simulink model "Aenea_model"  (R2020b)
settings: Solver=FixedStepDiscrete  StartTime=0.0  StopTime=10.0  FixedStep=0.02  RelTol=1e-3
values from neighbouring files (symbols this model uses):
  attuatore_Amax = deg2rad(27)    [AVVIO_AENEA_DATA.m]
  attuatore_Amin = deg2rad(-23)    [AVVIO_AENEA_DATA.m]
  attuatore_Emax = deg2rad(18)    [AVVIO_AENEA_DATA.m]
  attuatore_Emin = deg2rad(-32)    [AVVIO_AENEA_DATA.m]
  attuatore_Rmax = deg2rad(30)    [AVVIO_AENEA_DATA.m]
  attuatore_Rmin = deg2rad(-30)    [AVVIO_AENEA_DATA.m]
  attuatore_Tmax = 1    [AVVIO_AENEA_DATA.m]
  attuatore_Tmin = 0    [AVVIO_AENEA_DATA.m]
  interventoA_05 = 6    [AVVIO_AENEA_DATA.m]
  interventoA_1 = 2    [AVVIO_AENEA_DATA.m]
  interventoE_05 = 7.5    [AVVIO_AENEA_DATA.m]
  interventoE_1 = 3.2    [AVVIO_AENEA_DATA.m]
  interventoT = 0.1    [AVVIO_AENEA_DATA.m]
  inv_A = -1    [AVVIO_AENEA_DATA.m]
  inv_comp_h = -1    [AVVIO_AENEA_DATA.m]
  inv_E = 1    [AVVIO_AENEA_DATA.m]
  inv_R = 1    [AVVIO_AENEA_DATA.m]
  inv_T = 1    [AVVIO_AENEA_DATA.m]
  K_AW_B_AP_quota = 1000    [AVVIO_AENEA_DATA.m]
  K_AW_B_becc = -250    [AVVIO_AENEA_DATA.m]
  K_AW_B_imb = 0    [AVVIO_AENEA_DATA.m]
  K_AW_B_roll = 500    [AVVIO_AENEA_DATA.m]
  K_imb_inv = -1    [AVVIO_AENEA_DATA.m]
  Kd_h_app = 0.085    [AVVIO_AENEA_DATA.m]
  Kd_h_flare = 0.01    [AVVIO_AENEA_DATA.m]
  Ki_AP_quota_select = 0.014    [AVVIO_AENEA_DATA.m]
  Ki_AP_rotta = 0.03    [AVVIO_AENEA_DATA.m]
  Ki_AP_vel = 0.001*8    (= 0.008)    [AVVIO_AENEA_DATA.m]
  Ki_becch = -0.064065*10    (= -0.64065)    [AVVIO_AENEA_DATA.m]
  Ki_h_app = 0.055    [AVVIO_AENEA_DATA.m]
  Ki_h_cruise = 0.008    [AVVIO_AENEA_DATA.m]
  Ki_h_flare = 0.07    [AVVIO_AENEA_DATA.m]
  Ki_roll = 0.025*10    (= 0.25)    [AVVIO_AENEA_DATA.m]
  Kp_AP_quota_hold_h = 0.15    [AVVIO_AENEA_DATA.m]
  Kp_AP_quota_hold_l = 1    [AVVIO_AENEA_DATA.m]
  Kp_AP_quota_select = 0.014    [AVVIO_AENEA_DATA.m]
  Kp_AP_rotta = 0.7    [AVVIO_AENEA_DATA.m]
  Kp_AP_vel = 0.2692/8    (= 0.03365)    [AVVIO_AENEA_DATA.m]
  Kp_becch = -0.1918*10    (= -1.918)    [AVVIO_AENEA_DATA.m]
  Kp_comp_h = 0.035*15    (= 0.525)    [AVVIO_AENEA_DATA.m]
  Kp_h_app_max = 0.086    [AVVIO_AENEA_DATA.m]
  Kp_h_app_min = 0.01    [AVVIO_AENEA_DATA.m]
  Kp_h_cruise = 0.04    [AVVIO_AENEA_DATA.m]
  Kp_h_flare = 0.1    [AVVIO_AENEA_DATA.m]
  Kp_imb = -0.04*10    (= -0.4)    [AVVIO_AENEA_DATA.m]
  Kp_p = 0.025*5    (= 0.125)    [AVVIO_AENEA_DATA.m]
  Kp_q = -0.025*5    (= -0.125)    [AVVIO_AENEA_DATA.m]
  Kp_roll = 0.11*10    (= 1.1)    [AVVIO_AENEA_DATA.m]
  Kp_Rotta_ATO = 4    [AVVIO_AENEA_DATA.m]
  phi_max = deg2rad(30)    [AVVIO_AENEA_DATA.m]
  phi_min = deg2rad(-30)    [AVVIO_AENEA_DATA.m]
  safe_phi = 55    [AVVIO_AENEA_DATA.m]
  safe_V = 40    [AVVIO_AENEA_DATA.m]
  t_AP = 0.02    [AVVIO_AENEA_DATA.m]
  theta_max = deg2rad(15)    [AVVIO_AENEA_DATA.m]
  theta_min = deg2rad(-15)    [AVVIO_AENEA_DATA.m]
  time_alarm_SAFE = 1    [AVVIO_AENEA_DATA.m]
  V_max = 30    [AVVIO_AENEA_DATA.m]
  V_stall = 11    [AVVIO_AENEA_DATA.m]
  vel_wp1_al = 25    [AVVIO_AENEA_DATA.m]
  vel_wp2_al = 20    [AVVIO_AENEA_DATA.m]
undefined symbols (not defined in the file or in its folder): bias, DiscIntNeverNeededParam, Newton, Q1B, R1B, Raphson, Sensor_Offsets, tsamp, UP, vd_ini
libraries: simulink_extras x44, slpidlib x8, simulink x6, dspsigops x4, arduinolib x3, svdutilitieslib x3, aerolibtransform2sys x2, aerolibtransform2 x2, aerosimlib x2, cstblocks x1
(part 1 of 8)
settings Model: Creator=giampaolo  LastModifiedBy=david
settings SolverCC: PositivePriorityOrder=on
settings OptimizationCC: DefaultParameterBehavior=Inlined  EnhancedBackFolding=on  PassReuseOutputArgsAs=Individual arguments  ZeroExternalMemoryAtStartup=off  ZeroInternalMemoryAtStartup=off  MaxStackSize=64  OptimizeBlockOrder=speed  DifferentSizesBufferReuse=on  OptimizationCustomize=off  EfficientTunableParamExpr=on
settings DebuggingCC: ParameterTunabilityLossMsg=error
settings HardwareCC: ProdBitPerPointer=32  ProdBitPerSizeT=32  ProdBitPerPtrDiffT=32  ProdLargestAtomicInteger=Long  ProdLargestAtomicFloat=Double  ProdWordSize=32  ProdHWDeviceType=ARM Compatible->ARM Cortex-M  HardwareBoardFeatureSet=SoCBlockset
settings SFSimCC: MATLABDynamicMemAlloc=off
settings RTWCC: Description=Teensy EC Target  SystemTargetFile=teensy_ec.tlc  GenCodeOnly=on  GenerateMakefile=off  PackageName=teensy  TemplateMakefile=teensy_ec.tmf  CustomInclude=C:\Users\39339\Desktop\ProjectAenea\sfunctions  TargetLang=C++
settings CodeAppCC: ForceParamTrailComments=on  IgnoreCustomStorageClasses=off  OperatorAnnotations=on  SimulinkDataObjDesc=on  SFDataObjDesc=on  InsertBlockDesc=on
settings STFCustomTargetCC: TargetLangStandard=C++03 (ISO)  MultiwordLength=256  GenerateSampleERTMain=on  ModelReferenceCompliant=off  ConcurrentExecutionCompliant=off  CombineOutputUpdateFcns=on  ERTCustomFileBanners=on  SupportContinuousTime=off  SupportNonInlinedSFcns=off  RemoveResetFunc=on  SupportVariableSizeSignals=on  MATLABClassNameForMDSCustomization=Simulink.SoftwareTarget.ERTCustomization  CPPClassGenCompliant=off  GRTInterface=off  SystemTargetFile=teensy_ec.tlc
settings ERTTargetCC: TargetLangStandard=C++03 (ISO)  GenerateSampleERTMain=on  ModelReferenceCompliant=off  ParMdlRefBuildCompliant=off  CompOptLevelCompliant=off  ConcurrentExecutionCompliant=off  SupportVariableSizeSignals=on  ModelStepFunctionPrototypeControlCompliant=off  CPPClassGenCompliant=off  UseToolchainInfoCompliant=off  InlinedParameterPlacement=NonHierarchical  ERTCustomFileTemplate=teensy_ec_file_process.tlc  EnableUserReplacementTypes=on

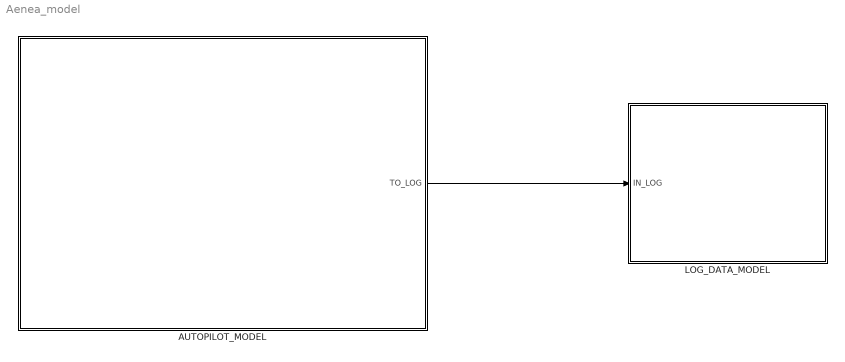
== system Aenea_model ==
  AUTOPILOT_MODEL : Subsystem  Priority=1
      settings: AttributesFormatString=priority = %<Priority>
  LOG_DATA_MODEL : Subsystem  Priority=2
      settings: AttributesFormatString=priority = %<Priority>
  wires:
  AUTOPILOT_MODEL/1(TO_LOG) -> LOG_DATA_MODEL/1(IN_LOG)

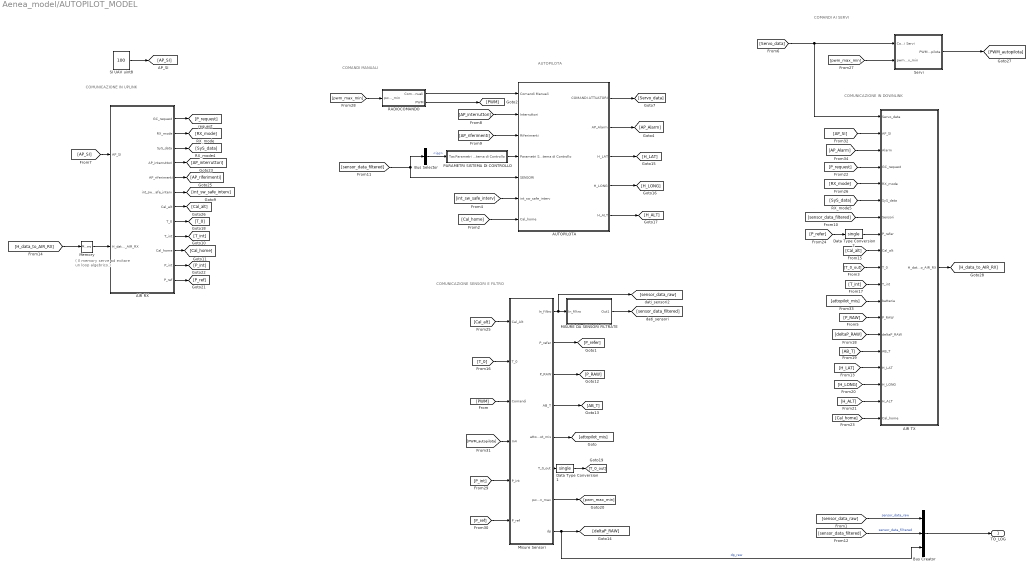
== system Aenea_model/AUTOPILOT_MODEL ==
  note: ( Il memory serve ad evitare
      | un loop algebrico.)
  note: COMUNICAZIONE IN DOWNLINK
  note: COMUNICAZIONE IN UPLINK
  note: COMUNICAZIONE SENSORI E FILTRO
  note: AUTOPILOTA
  note: COMANDI MANUALI
  note: COMANDI AI SERVI
  AIR RX : Subsystem
  AIR TX : Subsystem
  AUTOPILOTA : Subsystem
  Bus Creator : BusCreator  Inputs=3
  Bus Selector : BusSelector  OutputSignals=ias
  Data Type Conversion1 : DataTypeConversion  OutDataTypeStr=single
  Data Type Conversion2 : DataTypeConversion  OutDataTypeStr=single
  MISURE DA SENSORI FILTRATE : Subsystem
  Memory : Memory
  Misure Sensori : Subsystem
  PARAMETRI SISTEMA DI CONTROLLO : Subsystem
  RADIOCOMANDO : Subsystem
  SI UAV uint8 : Constant  Value=100  OutDataTypeStr=uint8
  Servi : Subsystem
  TO_LOG : Outport
  wires:
  [P_RAW] -> AIR TX/13(P_RAW)
  [T_int] -> AIR TX/11(T_int)
  [AP_SI] -> AIR RX/1(AP_SI)
  [AP_Alarm] -> AIR TX/3(Alarm)
  AIR RX/12(P_ref) -> [P_ref]
  [PWM] -> Misure Sensori/3(Comandi)
  AIR RX/5(AP_riferimenti) -> [AP_riferimenti]
  [RX_mode] -> AIR TX/5(RX_mode)
  AIR RX/7(Cal_alt) -> [Cal_alt]
  [Cal_home] -> AUTOPILOTA/7(Cal_home)
  MISURE DA SENSORI FILTRATE/1(Out1) -> [sensor_data_filtered]
  AIR RX/6(int_sw_safe_interv) -> [int_sw_safe_interv]
  AUTOPILOTA/3(H_LAT) -> [H_LAT]
  Memory/1 -> AIR RX/2(H_data_to_AIR_RX)
  [P_refer] -> Data Type Conversion2/1
  [AP_SI] -> AIR TX/2(AP_SI)
  Misure Sensori/7(pwm_min_max) -> [pwm_max_min]
  AIR RX/10(Cal_home) -> [Cal_home]
  [P_request] -> AIR TX/4(GC_request)
  [H_ALT] -> AIR TX/18(H_ALT)
  AIR RX/8(T_0) -> [T_0]
  [H_LONG] -> AIR TX/17(H_LONG)
  Servi/1(PWM_autopilota) -> [PWM_autopilota]
  AIR RX/1(GC_request) -> [P_request]
  [Servo_data] -> AIR TX/1(Servo_data), Servi/1(Comandi Servi)
  [AP_riferimenti] -> AUTOPILOTA/3(Riferimenti)
  [Cal_alt] -> Misure Sensori/1(Cal_Alt)
  Misure Sensori/5(attopilot_mis) -> [attopilot_mis]
  AIR RX/4(AP_interruttori) -> [AP_interruttori]
  [P_ref] -> Misure Sensori/6(P_ref)
  [sensor_data_filtered] -> Bus Selector/1, AUTOPILOTA/5(SENSORI)
  [attopilot_mis] -> AIR TX/12(batteria)
  [T_0_out] -> AIR TX/10(T_0)
  AIR RX/3(SyS_data) -> [SyS_data]
  SI UAV uint8/1 -> [AP_SI]
  [AP_interruttori] -> AUTOPILOTA/2("Interruttori ")
  AUTOPILOTA/1(COMANDI ATTUATORI) -> [Servo_data]
  AIR RX/11(P_int) -> [P_int]
  Bus Selector/1 -> PARAMETRI SISTEMA DI CONTROLLO/1(Tas)  "<ias>"
  Data Type Conversion1/1 -> [T_0_out]
  Misure Sensori/6(T_0_out) -> Data Type Conversion1/1
  [T_0] -> Misure Sensori/2(T_0)
  [sensor_data_filtered] -> AIR TX/7(Sensori)
  RADIOCOMANDO/1(Comandi Manuali) -> AUTOPILOTA/1(Comandi Manuali)
  [pwm_max_min] -> RADIOCOMANDO/1(pwm_max_min)
  [Cal_alt] -> AIR TX/9(Cal_alt)
  [Cal_home] -> AIR TX/19(Cal_home)
  Data Type Conversion2/1 -> AIR TX/8(P_refer)
  AIR RX/9(T_int) -> [T_int]
  AUTOPILOTA/5(H_ALT) -> [H_ALT]
  [deltaP_RAW] -> AIR TX/14(deltaP_RAW)
  [pwm_max_min] -> Servi/2(pwm_max_min)
  AUTOPILOTA/2(AP_Alarm) -> [AP_Alarm]
  Misure Sensori/3(P_RAW) -> [P_RAW]
  [H_data_to_AIR_RX] -> Memory/1
  Misure Sensori/1(In_filtro) -> [sensor_data_raw], MISURE DA SENSORI FILTRATE/1(In_filtro)
  PARAMETRI SISTEMA DI CONTROLLO/1(Parametri Sistema di Controllo) -> AUTOPILOTA/4(Parametri Sistema di Controllo)
  [H_LAT] -> AIR TX/16(H_LAT)
  [int_sw_safe_interv] -> AUTOPILOTA/6(int_sw_safe_interv)
  [SyS_data] -> AIR TX/6(SyS_data)
  [P_int] -> Misure Sensori/5(P_int)
  AIR TX/1(H_data_to_AIR_RX) -> [H_data_to_AIR_RX]
  Misure Sensori/2(P_refer) -> [P_refer]
  RADIOCOMANDO/2(PWM) -> [PWM]
  [AB_T] -> AIR TX/15(AB_T)
  [PWM_autopilota] -> Misure Sensori/4(In4)
  AIR RX/2(RX_mode) -> [RX_mode]
  Misure Sensori/4(AB_T) -> [AB_T]
  AUTOPILOTA/4(H_LONG) -> [H_LONG]
  [sensor_data_raw] -> Bus Creator/1  "sensor_data_raw"
  [sensor_data_filtered] -> Bus Creator/2  "sensor_data_filtered"
  Bus Creator/1 -> TO_LOG/1
  Misure Sensori/8(dp) -> Bus Creator/3, [deltaP_RAW]  "dp_raw"

== system Aenea_model/LOG_DATA_MODEL ==
  IN_LOG : Inport
  Bus Creator1 : BusCreator  Inputs=9  OutDataTypeStr=Bus: BUS_log_t  NonVirtualBus=on
      settings: InheritFromInputs=off
  Compare To Constant : simulink/Logic and Bit Operations/Compare To Constant  relop===  const=50  OutDataTypeStr=boolean
  Counter Limited : simulink/Sources/Counter Limited  uplimit=50  tsamp=-1
  LOG_BOOL_SIGNALS : Subsystem
  LOG_DOUBLE_SIGNALS : Subsystem
  LOG_INT16_SIGNALS : Subsystem
  LOG_INT32_SIGNALS : Subsystem
  LOG_INT8_SIGNALS : Subsystem
  LOG_SINGLE_SIGNALS : Subsystem
  LOG_UINT16_SIGNALS : Subsystem
  LOG_UINT32_SIGNALS : Subsystem
  LOG_UINT8_SIGNALS : Subsystem
  S-Function Builder : S-Function  FunctionName=Signal_Logger_sfun  SFunctionModules=Signal_Logger_sfun_wrapper  SFunctionDeploymentMode=off  EnableBusSupport=off  mask(S-Function Builder){}
      mask help: Simulink:masks:SFunctionBuilder_MD
      mask init:
      | val = [[.9  0.75 0.75 1 1 .9 .9 1]',[1 1 0.75 0.75 .9 .9 1 .9]'];try , sys = get_param(gcb,'SfunBuilderFcnName');if isempty(sys), sys = get_param(gcb,'FunctionName'); end,catch, sys = get_param(gcb,'FunctionName'); end
      settings: CopyFcn=set_param(gcbh,'LinkStatus','none')  OpenFcn=sfunctionwizard(gcbh)
      mask Display: plot(val(:,1),val(:,2)),disp(sys),port_label('input',1,'flightData'),port_label('input',2,'sec_flag')
  wires:
  Counter Limited/1 -> Compare To Constant/1
  Compare To Constant/1 -> LOG_BOOL_SIGNALS/1(dummy16), S-Function Builder/2  "dummy16"
  Bus Creator1/1 -> S-Function Builder/1
  LOG_BOOL_SIGNALS/1(bool_data) -> Bus Creator1/9
  LOG_UINT8_SIGNALS/1(uint8_data) -> Bus Creator1/8
  LOG_INT8_SIGNALS/1(int8_data) -> Bus Creator1/7
  LOG_UINT16_SIGNALS/1(uint16_data) -> Bus Creator1/6
  LOG_INT16_SIGNALS/1(int16_data) -> Bus Creator1/5
  LOG_UINT32_SIGNALS/1(uint32_data) -> Bus Creator1/4
  LOG_INT32_SIGNALS/1(int32_data) -> Bus Creator1/3
  LOG_SINGLE_SIGNALS/1(single_data) -> Bus Creator1/2
  IN_LOG/1 -> LOG_UINT8_SIGNALS/1(uint8_in), LOG_DOUBLE_SIGNALS/1(double_in), LOG_SINGLE_SIGNALS/1(single_in), LOG_INT16_SIGNALS/1(int16_in)
  LOG_DOUBLE_SIGNALS/1(double_data) -> Bus Creator1/1

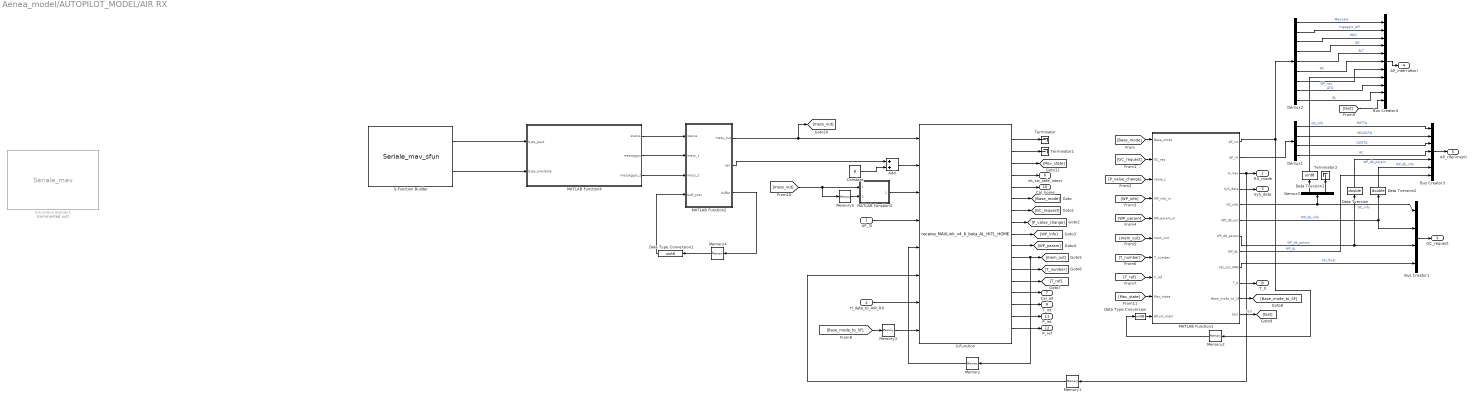
== system Aenea_model/AUTOPILOT_MODEL/AIR RX ==
  AP_SI : Inport
  H_data_to_AIR_RX : Inport  Port=2
  Add : Sum  AccumDataTypeStr=int32
  Bus Creator1 : BusCreator  Inputs=4
  Bus Creator3 : BusCreator  Inputs=7
  Bus Creator4 : BusCreator  Inputs=11
  Constant : Constant  Value=8  OutDataTypeStr=int32  SampleTime=-1
  Data Tversion : DataTypeConversion  OutDataTypeStr=double
  Data Tversion1 : DataTypeConversion  OutDataTypeStr=uint8
  Data Tversion2 : DataTypeConversion  OutDataTypeStr=double
  Data Type Conversion : DataTypeConversion  OutDataTypeStr=uint8
  Data Type Conversion1 : DataTypeConversion  OutDataTypeStr=uint8
  Demux1 : Demux
  Demux2 : Demux  Outputs=9
  Demux3 : Demux  Outputs=[1 2]
  MATLAB Function1 : MATLAB Function  TreatAsAtomicUnit=on
  MATLAB Function2 : MATLAB Function  TreatAsAtomicUnit=on
  MATLAB Function3 : MATLAB Function  TreatAsAtomicUnit=on
  MATLAB Function4 : MATLAB Function  TreatAsAtomicUnit=on
  Memory : Memory  InheritSampleTime=on
  Memory1 : Memory  InheritSampleTime=on
  Memory2 : Memory  InitialCondition=[0 0 0 0 0 0 0 0 0]
  Memory3 : Memory
  Memory4 : Memory  InitialCondition=uint8(zeros(3,100))  InheritSampleTime=on
  Memory5 : Memory  InheritSampleTime=on
  S-Function : S-Function  FunctionName=receive_MAVLink_v4_6_beta_AL_HITL_HOME  SFunctionModules='receive_MAVLink_v4_6_beta_AL_HITL_HOME_wrapper'  SFunctionDeploymentMode=off  EnableBusSupport=off
  S-Function Builder : S-Function  FunctionName=Seriale_mav_sfun  SFunctionModules=Seriale_mav_sfun_wrapper  SFunctionDeploymentMode=off  EnableBusSupport=off  mask(S-Function Builder){}
      mask help: Simulink:masks:SFunctionBuilder_MD
      mask init: same as Aenea_model/LOG_DATA_MODEL/S-Function Builder
      settings: CopyFcn=set_param(gcbh,'LinkStatus','none')  OpenFcn=sfunctionwizard(gcbh)
      mask Display: plot(val(:,1),val(:,2)),disp(sys),port_label('output',1,'Messaggio'),port_label('output',2,'serial_available')
  S-Function Builder1 : S-Function  Commented=on  InitFcn=try, set_param(gcb,'FunctionName','Seriale_mav'), end  FunctionName=Seriale_mav  SFunctionModules=Seriale_mav_wrapper  SFunctionDeploymentMode=off  EnableBusSupport=off  mask(S-Function Builder){}
      mask help: Simulink:masks:SFunctionBuilder_MD
      mask init: same as Aenea_model/LOG_DATA_MODEL/S-Function Builder
      settings: CopyFcn=set_param(gcbh,'LinkStatus','none')  PreSaveFcn=try, set_param(gcb,'FunctionName','Seriale_mav'), end  OpenFcn=sfunctionwizard(gcbh)
      mask Display: plot(val(:,1),val(:,2)),disp(sys),port_label('output',1,'Messaggio'),port_label('output',2,'serial_available')
  Terminator : Terminator
  Terminator1 : Terminator
  Terminator2 : Terminator
  GC_request : Outport  VectorParamsAs1DForOutWhenUnconnected=off
  RX_mode : Outport  Port=2  VectorParamsAs1DForOutWhenUnconnected=off
  SyS_data : Outport  Port=3  VectorParamsAs1DForOutWhenUnconnected=off
  AP_interruttori : Outport  Port=4  VectorParamsAs1DForOutWhenUnconnected=off
  AP_riferimenti : Outport  Port=5  VectorParamsAs1DForOutWhenUnconnected=off
  int_sw_safe_interv : Outport  Port=6  VectorParamsAs1DForOutWhenUnconnected=off
  Cal_alt : Outport  Port=7  VectorParamsAs1DForOutWhenUnconnected=off
  T_0 : Outport  Port=8  VectorParamsAs1DForOutWhenUnconnected=off
  T_int : Outport  Port=9  VectorParamsAs1DForOutWhenUnconnected=off
  Cal_home : Outport  Port=10  VectorParamsAs1DForOutWhenUnconnected=off
  P_int : Outport  Port=11  VectorParamsAs1DForOutWhenUnconnected=off
  P_ref : Outport  Port=12  VectorParamsAs1DForOutWhenUnconnected=off
  wires:
  H_data_to_AIR_RX/1 -> S-Function/7
  Memory1/1 -> S-Function/6
  Memory/1 -> S-Function/5
  Memory3/1 -> S-Function/8
  AP_SI/1 -> S-Function/4
  Demux2/6 -> Bus Creator4/6  "RC"
  Data Tversion1/1 -> Bus Creator4/8  "GC_info"
  Memory2/1 -> Data Type Conversion/1
  Bus Creator1/1 -> GC_request/1
  Demux1/2 -> Bus Creator3/2  "VELOCITA"
  Demux2/5 -> Bus Creator4/5  "ALT"
  Demux2/1 -> Bus Creator4/1  "Manuale"
  Demux2/3 -> Bus Creator4/3  "HDG"
  [P_value_change] -> MATLAB Function1/3(value_c)
  Demux1/4 -> Bus Creator3/4  "RC"
  MATLAB Function1/2(AP_rif) -> Demux1/1
  Demux2/8 -> Bus Creator4/9  "ATO"
  MATLAB Function1/7(WP_db_param) -> Bus Creator1/3, Data Tversion/1  "WP_db_param"
  [GC_request] -> MATLAB Function1/2(GC_req)
  Demux2/2 -> Bus Creator4/2  "Ingaggio_A/P"
  [mem_out] -> MATLAB Function1/6(mem_out)
  Bus Creator4/1 -> AP_interruttori/1
  MATLAB Function1/4(SyS_data) -> SyS_data/1
  MATLAB Function1/6(WP_db_out) -> Data Tversion2/1, Bus Creator1/2  "WP_db_info"
  [Mav_state] -> MATLAB Function1/9(Mav_state)
  Demux2/7 -> Bus Creator4/7  "WP_nav"
  [T_ref] -> MATLAB Function1/8(T_ref)
  Data Type Conversion/1 -> MATLAB Function1/10(AP_int_mem)
  Data Tversion2/1 -> Bus Creator3/6  "WP_db_info"
  Demux3/2 -> Terminator2/1
  [Base_mode] -> MATLAB Function1/1(Base_mode)
  [WP_param] -> MATLAB Function1/5(WP_param_in)
  Data Tversion/1 -> Bus Creator3/5  "WP_db_param"
  Demux3/1 -> Data Tversion1/1
  MATLAB Function1/3(H_mav) -> Memory1/1, RX_mode/1
  MATLAB Function1/9(Val_out_MAV) -> Bus Creator1/4  "Val_float"
  Bus Creator3/1 -> AP_riferimenti/1
  [T_number] -> MATLAB Function1/7(T_number)
  MATLAB Function1/5(GC_info) -> Demux3/1, Bus Creator1/1  "GC_info"
  MATLAB Function1/1(AP_int) -> Demux2/1, Memory2/1
  [WP_info] -> MATLAB Function1/4(WP_info_in)
  [Base_mode_to_SF] -> Memory3/1
  MATLAB Function1/11(Base_mode_to_SF) -> [Base_mode_to_SF]
  Demux1/3 -> Bus Creator3/3  "QUOTA"
  MATLAB Function1/12(test) -> [test]  "test"
  Demux2/4 -> Bus Creator4/4  "IAS"
  [test] -> Bus Creator4/11
  Demux1/1 -> Bus Creator3/1  "ROTTA"
  MATLAB Function1/8(WP_AL) -> Bus Creator3/7  "WP_AL"
  MATLAB Function1/10(T_0) -> T_0/1
  Demux2/9 -> Bus Creator4/10  "AL"
  MATLAB Function4/3(messaggio_2) -> MATLAB Function2/3(mess_2)
  MATLAB Function2/2(Len) -> Add/1
  MATLAB Function4/1(status) -> MATLAB Function2/1(status)
  MATLAB Function4/2(messaggio) -> MATLAB Function2/2(mess_1)
  Memory4/1 -> Data Type Conversion1/1
  MATLAB Function2/3(buffer) -> Memory4/1
  Constant/1 -> Add/2
  MATLAB Function2/1(mess_out) -> S-Function/1, [mess_out]
  Add/1 -> S-Function/2
  Data Type Conversion1/1 -> MATLAB Function2/4(buff_prev)
  Memory5/1 -> MATLAB Function3/2(mess_out_prev)
  [mess_out] -> Memory5/1, MATLAB Function3/1(mess_out)
  MATLAB Function3/1(new_mex) -> S-Function/3
  S-Function/1 -> Terminator/1
  S-Function/2 -> Terminator1/1
  S-Function/3 -> [Mav_state]
  S-Function/4 -> int_sw_safe_interv/1
  S-Function/5 -> Cal_home/1
  S-Function/6 -> [Base_mode]
  S-Function/7 -> [GC_request]
  S-Function/8 -> [P_value_change]
  S-Function/9 -> [WP_info]
  S-Function/10 -> [WP_param]
  S-Function/11 -> Memory/1, [mem_out]
  S-Function/12 -> [T_number]
  S-Function/13 -> [T_ref]
  S-Function/14 -> Cal_alt/1
  S-Function/15 -> T_int/1
  S-Function/16 -> P_int/1
  S-Function/17 -> P_ref/1
  S-Function Builder/1 -> MATLAB Function4/1(byte_pack)
  S-Function Builder/2 -> MATLAB Function4/2(byte_available)

== system Aenea_model/AUTOPILOT_MODEL/AIR TX ==
  Servo_data : Inport
  AP_SI : Inport  Port=2
  Alarm : Inport  Port=3
  GC_request : Inport  Port=4
  RX_mode : Inport  Port=5
  SyS_data : Inport  Port=6
  Sensori : Inport  Port=7
  P_refer : Inport  Port=8
  Cal_alt : Inport  Port=9
  T_0 : Inport  Port=10
  T_int : Inport  Port=11
  batteria : Inport  Port=12
  P_RAW : Inport  Port=13
  deltaP_RAW : Inport  Port=14
  AB_T : Inport  Port=15
  H_LAT : Inport  Port=16
  H_LONG : Inport  Port=17
  H_ALT : Inport  Port=18
  Cal_home : Inport  Port=19
  Data Type Conversion : DataTypeConversion  OutDataTypeStr=single
  Data Type Conversion1 : DataTypeConversion  OutDataTypeStr=single
  Data Type Conversion2 : DataTypeConversion  OutDataTypeStr=int16
  "Enable " : Subsystem  Commented=on  TreatAsAtomicUnit=on
  GPS : Subsystem  SystemSampleTime=0.02
  Ground : Ground
  Heartbeat : Subsystem  SystemSampleTime=1
  IMU & Attidude : Subsystem  SystemSampleTime=0.04
  If_subsystem : Subsystem
  Memory : Memory
  Pa to hPa : Gain  Gain=0.01
  Pa to hPa1 : Gain  Gain=0.01
  S-Function : S-Function  FunctionName=send_MAVLink_v4_4_2_beta_3_HOME  SFunctionModules='send_MAVLink_v4_4_2_beta_3_HOME_wrapper'  SFunctionDeploymentMode=off  EnableBusSupport=off
  S-Function Builder : S-Function  FunctionName=enable_sfun  SFunctionModules=enable_sfun_wrapper  SFunctionDeploymentMode=off  EnableBusSupport=off  mask(S-Function Builder){}
      mask help: Simulink:masks:SFunctionBuilder_MD
      mask init: same as Aenea_model/LOG_DATA_MODEL/S-Function Builder
      settings: CopyFcn=set_param(gcbh,'LinkStatus','none')  OpenFcn=sfunctionwizard(gcbh)
      mask Display: plot(val(:,1),val(:,2)),disp(sys),port_label('input',1,'u0'),port_label('output',1,'y0')
  Servo : Subsystem  SystemSampleTime=0.5
  Subsystem : Subsystem
  SystemStatus : Subsystem  SystemSampleTime=0.2
  VFR : Subsystem  SystemSampleTime=0.5
  Waypoints : Subsystem  SystemSampleTime=1
  H_data_to_AIR_RX : Outport  VectorParamsAs1DForOutWhenUnconnected=off
  wires:
  Alarm/1 -> SystemStatus/2(Alarm), Heartbeat/1(Alarm)
  RX_mode/1 -> Heartbeat/2(RX_mode)
  deltaP_RAW/1 -> Pa to hPa1/1
  Sensori/1 -> Waypoints/2("Sensori "), Servo/1(Sensor), VFR/1(VFR1), GPS/1(GPS1), IMU & Attidude/1(AHRS1)
  SyS_data/1 -> SystemStatus/1(SyS_input)
  GC_request/1 -> Waypoints/1(GC_req)
  Servo_data/1 -> Servo/2(Servo)
  AB_T/1 -> Data Type Conversion2/1
  Pa to hPa/1 -> Data Type Conversion/1
  P_RAW/1 -> Pa to hPa/1
  Pa to hPa1/1 -> Data Type Conversion1/1
  batteria/1 -> SystemStatus/3(batteria)
  S-Function/2 -> Subsystem/1(In1)
  S-Function/3 -> Subsystem/2(In2)
  S-Function/1 -> S-Function Builder/1
  If_subsystem/1(iflogic) -> S-Function/1
  If_subsystem/2(time) -> S-Function/2
  AP_SI/1 -> S-Function/3
  Waypoints/1(GC_info) -> S-Function/4
  Waypoints/2(P_value) -> S-Function/5
  Waypoints/3(WP_info) -> S-Function/6
  Waypoints/4(WP_param) -> S-Function/7
  SystemStatus/1(onboard) -> S-Function/8
  SystemStatus/2(LVDE) -> S-Function/9
  SystemStatus/3(B_current) -> S-Function/10
  SystemStatus/4(B_remaining) -> S-Function/11
  Heartbeat/1(custom) -> S-Function/12
  Heartbeat/2(H_data) -> H_data_to_AIR_RX/1, S-Function/13
  IMU & Attidude/1(IMU) -> S-Function/14
  IMU & Attidude/2(ATT) -> S-Function/15
  GPS/1(LLAA) -> S-Function/16
  GPS/2(vel) -> S-Function/17
  GPS/3(hdg1) -> S-Function/18
  VFR/1(AGAC) -> S-Function/19
  VFR/2(Heading) -> S-Function/20
  VFR/3(Throttle) -> S-Function/21
  Servo/1(Servo_data) -> S-Function/22
  P_refer/1 -> S-Function/24
  Cal_alt/1 -> S-Function/25
  T_0/1 -> S-Function/26
  T_int/1 -> S-Function/27
  Data Type Conversion/1 -> S-Function/28
  Data Type Conversion1/1 -> S-Function/29
  Data Type Conversion2/1 -> S-Function/30
  Cal_home/1 -> S-Function/31
  H_LAT/1 -> S-Function/32
  H_LONG/1 -> S-Function/33
  H_ALT/1 -> S-Function/34
  Ground/1 -> S-Function/35
  S-Function/4 -> Memory/1
  Memory/1 -> S-Function/23
  S-Function Builder/1 -> Subsystem/Enable

== system Aenea_model/AUTOPILOT_MODEL/AUTOPILOTA ==
  note: SISTEMA DI GESTIONE
  note: LOOP INTERNI e SWITCH
  note: MODI A/P
  note: LOOP ESTERNI e SWITCH
  Comandi Manuali : Inport
  "Interruttori " : Inport  Port=2
  Riferimenti : Inport  Port=3
  Parametri Sistema di Controllo : Inport  Port=4
  SENSORI : Inport  Port=5
  int_sw_safe_interv : Inport  Port=6
  Cal_home : Inport  Port=7
  AUTOPILOTI1 : Subsystem
  CONTROLLI INTERNI E SWITCH1 : Subsystem
  Demux : Demux  Outputs=2
  GESTIONE AUTOPILOTI1 : Subsystem
  Mux : Mux  Inputs=2
  Subsystem1 : Subsystem
  Terminator : Terminator
  COMANDI ATTUATORI : Outport  VectorParamsAs1DForOutWhenUnconnected=off
  AP_Alarm : Outport  Port=2  VectorParamsAs1DForOutWhenUnconnected=off
  H_LAT : Outport  Port=3  VectorParamsAs1DForOutWhenUnconnected=off
  H_LONG : Outport  Port=4  VectorParamsAs1DForOutWhenUnconnected=off
  H_ALT : Outport  Port=5  VectorParamsAs1DForOutWhenUnconnected=off
  wires:
  AUTOPILOTI1/1(Riferimento Manetta) -> CONTROLLI INTERNI E SWITCH1/3(Riferimento Manetta)
  Subsystem1/4(Riferimenti) -> AUTOPILOTI1/3(Riferimenti)
  GESTIONE AUTOPILOTI1/6(Switch_ATO) -> [Switch_ATO]
  Subsystem1/2(H_LONG) -> H_LONG/1
  GESTIONE AUTOPILOTI1/5(Alarm Safe) -> AUTOPILOTI1/5(Alarm Safe), Mux/1
  Demux/1 -> GESTIONE AUTOPILOTI1/4(int_sw_safe)
  GESTIONE AUTOPILOTI1/3(modo) -> Subsystem1/4(modo)
  [Switch_ATO] -> AUTOPILOTI1/8(Switch_ATO)
  "Interruttori "/1 -> GESTIONE AUTOPILOTI1/2("Interruttori "), Subsystem1/2(Interruttori)
  [Switch_AL] -> AUTOPILOTI1/9(Switch_AL)
  [Switch_ATO] -> CONTROLLI INTERNI E SWITCH1/6(Switch_ATO)
  Mux/1 -> AP_Alarm/1
  Cal_home/1 -> Subsystem1/5(Cal_home)
  GESTIONE AUTOPILOTI1/1(Switch Attuatori) -> Subsystem1/6(Switch_attuatori), AUTOPILOTI1/7(Switch attuatori), CONTROLLI INTERNI E SWITCH1/4(Switch Attuatori)
  CONTROLLI INTERNI E SWITCH1/3(manetta_track) -> AUTOPILOTI1/11(manetta_track)
  Comandi Manuali/1 -> AUTOPILOTI1/6(comandi), CONTROLLI INTERNI E SWITCH1/2(Comandi Manuali), GESTIONE AUTOPILOTI1/3(Comandi Manuali)
  GESTIONE AUTOPILOTI1/7(Switch_AL) -> [Switch_AL]
  CONTROLLI INTERNI E SWITCH1/2(theta_track) -> AUTOPILOTI1/10(traking theta)
  CONTROLLI INTERNI E SWITCH1/4(phi_track) -> AUTOPILOTI1/12(track_phi)
  AUTOPILOTI1/2(Riferimenti Rollio e Beccheggio) -> Terminator/1
  Parametri Sistema di Controllo/1 -> AUTOPILOTI1/2(Parametri Sistema di Controllo), CONTROLLI INTERNI E SWITCH1/1(Parametri Sistema di Controllo)
  Demux/2 -> GESTIONE AUTOPILOTI1/5(int_sw_intervento)
  GESTIONE AUTOPILOTI1/4(Alarm Intervento) -> Mux/2
  [Switch_AL] -> CONTROLLI INTERNI E SWITCH1/7(Switch_AL)
  int_sw_safe_interv/1 -> Demux/1
  CONTROLLI INTERNI E SWITCH1/1(Comandi Attuatori) -> COMANDI ATTUATORI/1
  Subsystem1/1(H_LAT) -> H_LAT/1
  GESTIONE AUTOPILOTI1/2(Riferimenti Safe) -> AUTOPILOTI1/4(Riferimenti Safe)
  Riferimenti/1 -> Subsystem1/3(waypoints e riferimenti vettoriali)
  SENSORI/1 -> GESTIONE AUTOPILOTI1/1(Sensori), Subsystem1/1(sensori), AUTOPILOTI1/1(Sensori), CONTROLLI INTERNI E SWITCH1/5(Sensori)
  Subsystem1/3(H_ALT) -> H_ALT/1
  Subsystem1/5(Inner_loop_ATO) -> CONTROLLI INTERNI E SWITCH1/8(Inner_loop_ATO)

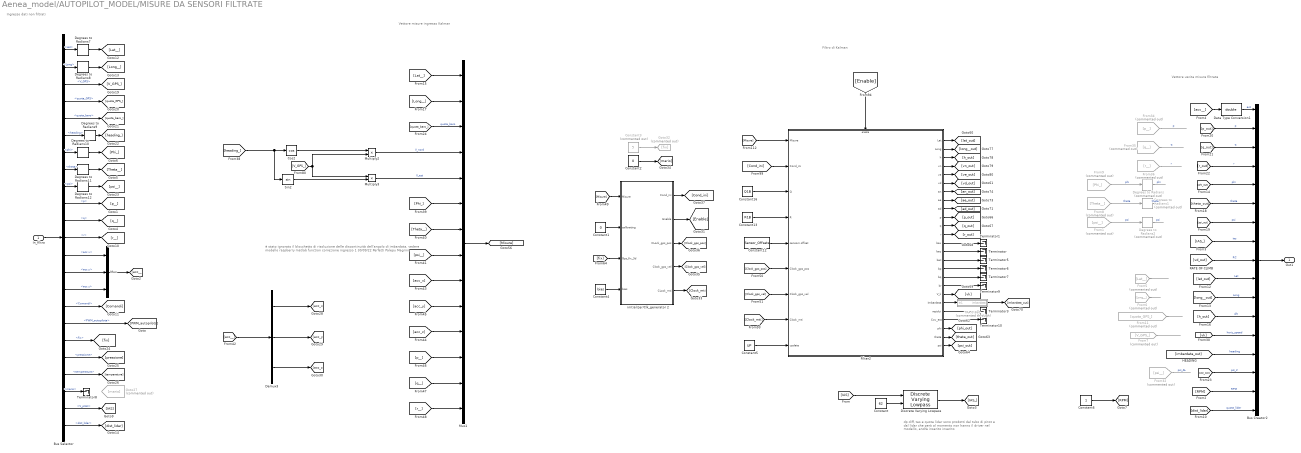
== system Aenea_model/AUTOPILOT_MODEL/MISURE DA SENSORI FILTRATE ==
  note: dp diff, tas e quota lidar
      |  sono prodotti dal tubo di pitot e dal lidar che però al momento non hanno il driver nel modello, andrà inserito inserito
  note: Vettore uscita misure filtrate
  note: Filtro di Kalman
  note: Vettore misure ingresso
      | Kalman
  note: Ingresso dati non filtrati
  note: è stato ignorato il blocchetto di risoluzione delle discontinuità dell'angolo di imbardata, vedere modello raspberry matlab function correzione ingresso 1 30/09/22 Perfetti Palepu Magrini
  In_filtro : Inport
  Bus Creator2 : BusCreator  Inputs=17
  Bus Selector : BusSelector  OutputSignals=Lat,Long,V_GPS,quota_GPS,quota_baro,heading,phi,theta,psi,p,q,r,acc x,acc y,acc z,Comandi,PWM_autopilota,fix,pressione,temperatura,mario,V_pitot,dist_lidar
  Constant : Constant  Value=62
  Constant1 : Constant  Value=0
  Constant12 : Constant  Value=Sensor_Offsets
  Constant13 : Constant  Value=R1B
  Constant16 : Constant  Value=Q1B
  Constant2 : Constant  Value=0
  Constant3 : Constant  Commented=on  Value=5
  Constant4 : Constant  Value=bias
  Constant5 : Constant  Value=UP
  Constant6 : Constant
  Cos2 : Trigonometry  Operator=cos
  Data Type Conversion1 : DataTypeConversion  OutDataTypeStr=double
  Degrees to Radians : simulink_extras/Transformations/Degrees to Radians  Commented=on
  Degrees to Radians1 : simulink_extras/Transformations/Degrees to Radians  Commented=on
  Degrees to Radians{7..12} (6 alike) : simulink_extras/Transformations/Degrees to Radians
  Degrees to Radians2 : simulink_extras/Transformations/Degrees to Radians  Commented=on
  Demux3 : Demux  Outputs=3
  Discrete Varying Lowpass : cstblocks/Linear Parameter Varying/Discrete Varying Lowpass  N=1  w0=0  Ts=t_AP
      settings: SourceProductBaseCode=CT
  Filter2 : Subsystem
  From1 : From  Commented=on  GotoTag=psi__
  From11 : From  Commented=on  GotoTag=quota_GPS_
  From32 : From  Commented=on  GotoTag=psi__
  From34 : From  Commented=on  GotoTag=p__
  From35 : From  Commented=on  GotoTag=q__
  From36 : From  Commented=on  GotoTag=r__
  From5 : From  Commented=on  GotoTag=Lat__
  From6 : From  Commented=on  GotoTag=Long__
  From7 : From  Commented=on  GotoTag=V_GPS_
  From8 : From  Commented=on  GotoTag=Theta__
  From9 : From  Commented=on  GotoTag=Phi_
  Goto27 : Goto  Commented=on  GotoTag=mario
  Goto32 : Goto  Commented=on  GotoTag=fix
  Multiply2 : Product
  Multiply3 : Product
  Mux : Mux  Inputs=3
  Mux1 : Mux  Inputs=14
  Sin2 : Trigonometry
  TRA 0-360 : Subsystem  Commented=through
  Terminator{,1,3,5..10} (9 alike) : Terminator
  initializer/Clk_generator 2 : Subsystem
  Out1 : Outport  VectorParamsAs1DForOutWhenUnconnected=off
  wires:
  From9/1 -> Degrees to Radians/1  "phi"
  Bus Selector/11 -> [q__]  "<q>"
  Bus Selector/7 -> Degrees to Radians10/1  "<phi>"
  Bus Selector/14 -> Mux/2  "<acc y>"
  From36/1 -> ?  "r"
  Bus Selector/10 -> [p__]  "<p>"
  Mux/1 -> [acc__]
  Bus Selector/13 -> Mux/1  "<acc x>"
  [vd_out] -> Bus Creator2/9  "RC"
  Bus Selector/12 -> [r__]  "<r>"
  Degrees to Radians/1 -> ?  "phi"
  From34/1 -> ?  "p"
  Bus Selector/5 -> [quota_baro_]  "<quota_baro>"
  Bus Selector/16 -> [Comandi]  "<Comandi>"
  Bus Selector/6 -> Degrees to Radians9/1  "<heading>"
  Bus Selector/3 -> [V_GPS_]  "<V_GPS>"
  Bus Selector/9 -> Degrees to Radians12/1  "<psi>"
  Bus Selector/15 -> Mux/3  "<acc z>"
  From1/1 -> Degrees to Radians2/1  "psi"
  From8/1 -> Degrees to Radians1/1  "theta"
  [vk] -> Bus Creator2/13  "horiz_speed"
  Bus Selector/1 -> Degrees to Radians7/1  "<Lat>"
  Bus Selector/19 -> [pressione]  "<pressione>"
  [imbardata_out] -> Bus Creator2/14  "heading"
  From35/1 -> ?  "q"
  Degrees to Radians1/1 -> ?  "theta"
  Bus Creator2/1 -> Out1/1
  [IAS_] -> Bus Creator2/8  "ias"
  [RPM] -> Bus Creator2/16  "RPM"
  Data Type Conversion1/1 -> Bus Creator2/1  "acc"
  Bus Selector/4 -> [quota_GPS_]  "<quota_GPS>"
  Bus Selector/18 -> [fix]  "<fix>"
  In_filtro/1 -> Bus Selector/1
  [acc__] -> Data Type Conversion1/1
  Bus Selector/20 -> [temperatura]  "<temperatura>"
  Bus Selector/21 -> Terminator8/1  "<mario>"
  Degrees to Radians2/1 -> ?  "psi"
  Bus Selector/8 -> Degrees to Radians11/1  "<theta>"
  [long__out] -> Bus Creator2/11  "Long"
  [h_out] -> Bus Creator2/12  "Alt"
  From32/1 -> ?  "psi_AL"
  [lat_out] -> Bus Creator2/10  "Lat"
  [dist_lidar] -> Bus Creator2/17  "quota_lidar"
  Bus Selector/2 -> Degrees to Radians8/1  "<Long>"
  Bus Selector/17 -> [PWM_autopilota]  "<PWM_autopilota>"
  [quota_baro_] -> Mux1/3  "quota_baro"
  Cos2/1 -> Multiply2/1
  [V_GPS_] -> Multiply2/2, Multiply3/1
  Multiply3/1 -> Mux1/5  "V_est"
  Multiply2/1 -> Mux1/4  "V_nord"
  Sin2/1 -> Multiply3/2
  [acc__] -> Demux3/1
  Demux3/3 -> [acc_z]
  Demux3/2 -> [acc_y]
  Demux3/1 -> [acc_x]
  [acc_z] -> Mux1/11
  [acc_y] -> Mux1/10
  [acc_x] -> Mux1/9
  [p__] -> Mux1/12
  [q__] -> Mux1/13
  [r__] -> Mux1/14
  [fix] -> initializer/Clk_generator 2/3(Gps_fix_3d)
  initializer/Clk_generator 2/5(CLock_mti) -> [Clock_mti]
  Constant3/1 -> Goto32/1
  initializer/Clk_generator 2/2(Enable) -> [Enable]
  Constant1/1 -> initializer/Clk_generator 2/2(calibrating)
  initializer/Clk_generator 2/3(CLock_gps_pos) -> [Clock_gps_pos]
  Filter2/3(h) -> [h_out]
  Constant4/1 -> initializer/Clk_generator 2/4(bias)
  Filter2/25(psi) -> [psi_out]
  Filter2/6(vd) -> [vd_out]
  Constant13/1 -> Filter2/4(R)
  Filter2/10(p) -> [p_out]
  Filter2/18(br) -> Terminator9/1
  Filter2/23(phi) -> [phi_out]
  Filter2/14(bay) -> Terminator/1
  [Cond_ini] -> Filter2/2(Cond_ini)
  Filter2/7(an) -> [an_out]
  Filter2/12(r) -> [r_out]
  initializer/Clk_generator 2/1(Cond_ini) -> [Cond_ini]
  Filter2/24(theta) -> [theta_out]
  Filter2/11(q) -> [q_out]
  initializer/Clk_generator 2/4("Clock_gps_vel ") -> [Clock_gps_vel]
  [Misure] -> initializer/Clk_generator 2/1(Misure)
  Filter2/2(Long) -> [long__out]
  Filter2/8(ae) -> [ae_out]
  Filter2/16(bp) -> Terminator6/1
  Filter2/9(ad) -> [ad_out]
  Filter2/4(vn) -> [vn_out]
  Constant16/1 -> Filter2/3(Q)
  Filter2/22(Cov_est) -> Terminator10/1
  Filter2/17(bq) -> Terminator7/1
  Filter2/21(residui) -> Terminator3/1
  [Clock_gps_vel] -> Filter2/7(Clock_gps_vel)
  Filter2/1(Lat) -> [lat_out]
  Filter2/15(baz) -> Terminator5/1
  [Enable] -> Filter2/Enable
  Constant2/1 -> [mario]
  Filter2/19(V_k) -> [vk]
  Filter2/20(Imbardata) -> TRA 0-360/1(In1)
  Constant12/1 -> Filter2/5(sensors offset)
  Filter2/13(bax) -> Terminator1/1
  Filter2/5(ve) -> [ve_out]
  Constant5/1 -> Filter2/9(update)
  [Misure] -> Filter2/1(Misure)
  [Clock_gps_pos] -> Filter2/6(Clock_gps_pos)
  TRA 0-360/1(imbardata) -> [imbardata_out]
  [Clock_mti] -> Filter2/8(Clock_mti)
  Mux1/1 -> [Misure]
  Constant/1 -> Discrete Varying Lowpass/2
  [IAS] -> Discrete Varying Lowpass/1
  Discrete Varying Lowpass/1 -> [IAS_]
  Constant6/1 -> [RPM]
  Bus Selector/22 -> [IAS]  "<V_pitot>"
  Bus Selector/23 -> [dist_lidar]  "<dist_lidar>"
  From5/1 -> ?
  From6/1 -> ?
  From7/1 -> ?
  From11/1 -> ?
  [Phi_] -> Mux1/6
  [Theta__] -> Mux1/7
  [psi__] -> Mux1/8
  [Lat__] -> Mux1/1
  [Long__] -> Mux1/2
  [heading_] -> Sin2/1, Cos2/1
  [psi_out] -> Bus Creator2/7  "psi"
  [theta_out] -> Bus Creator2/6  "theta"
  [phi_out] -> Bus Creator2/5  "phi"
  [p_out] -> Bus Creator2/2  "p"
  [q_out] -> Bus Creator2/3  "q"
  [r_out] -> Bus Creator2/4  "r"
  [psi_out] -> Bus Creator2/15  "psi_2"
  Degrees to Radians10/1 -> [Phi_]
  Degrees to Radians11/1 -> [Theta__]
  Degrees to Radians12/1 -> [psi__]
  Degrees to Radians7/1 -> [Lat__]
  Degrees to Radians8/1 -> [Long__]
  Degrees to Radians9/1 -> [heading_]

== system Aenea_model/AUTOPILOT_MODEL/Misure Sensori ==
  Cal_Alt : Inport
  T_0 : Inport  Port=2
  Comandi : Inport  Port=3
  In4 : Inport  Port=4
  P_int : Inport  Port=5
  P_ref : Inport  Port=6
  ATTOPILOT : Subsystem  Commented=on
  BMP_280 : Subsystem
  Bus Creator : BusCreator  Inputs=23
  Byte Unpack : svdutilitieslib/Byte Unpack  dimensions={[8]}  datatypes={'uint16'}  byteAlign=1  blockPlatform=arduinoert
      settings: SourceProductBaseCode=ARDUINO
  Compare To Constant : simulink/Logic and Bit Operations/Compare To Constant  relop===  const=1  OutDataTypeStr=boolean
  Constant : Constant  Value=[0 0 0]
  Constant1 : Constant  Value=[1,2,3,4,5,6,7,8,9]
  Constant2 : Constant  Value=0
  Constant3 : Constant  Value=0
  Constant8 : Constant  Value=[23,24,25,26,27,28]
  Constant9 : Constant  Value=29
  Counter Limited : simulink/Sources/Counter Limited  uplimit=1  tsamp=1
  Data Type Conversion1 : DataTypeConversion  OutDataTypeStr=double
  Demux : Demux  Outputs=6
  Demux1 : Demux  Outputs=9
  GPS_Venus : Subsystem
  MTi : Subsystem
  Manual Switch : ManualSwitch
  Manual Switch1 : ManualSwitch  CurrentSetting=0
  Manual Switch2 : ManualSwitch
  Manual Switch3 : ManualSwitch  CurrentSetting=0
  Pitot_Lidar : Subsystem
  S-Function Builder : S-Function  FunctionName=blink_sfun  SFunctionModules=blink_sfun_wrapper  SFunctionDeploymentMode=off  EnableBusSupport=off  mask(S-Function Builder){}
      mask help: Simulink:masks:SFunctionBuilder_MD
      mask init: same as Aenea_model/LOG_DATA_MODEL/S-Function Builder
      settings: CopyFcn=set_param(gcbh,'LinkStatus','none')  OpenFcn=sfunctionwizard(gcbh)
      mask Display: plot(val(:,1),val(:,2)),disp(sys),port_label('input',1,'clock')
  registro memoria2 13 : Constant  Value=ones(16,1)  OutDataTypeStr=uint8  SampleTime=t_AP
  In_filtro : Outport  VectorParamsAs1DForOutWhenUnconnected=off
  P_refer : Outport  Port=2  VectorParamsAs1DForOutWhenUnconnected=off
  P_RAW : Outport  Port=3  VectorParamsAs1DForOutWhenUnconnected=off
  AB_T : Outport  Port=4  VectorParamsAs1DForOutWhenUnconnected=off
  attopilot_mis : Outport  Port=5  VectorParamsAs1DForOutWhenUnconnected=off
  T_0_out : Outport  Port=6  VectorParamsAs1DForOutWhenUnconnected=off
  pwm_min_max : Outport  Port=7  VectorParamsAs1DForOutWhenUnconnected=off
  dp : Outport  Port=8
  wires:
  Demux1/8 -> Bus Creator/15  "theta"
  Demux/6 -> Bus Creator/6  "fix"
  GPS_Venus/1(Misure_GPS1) -> Manual Switch/1
  P_ref/1 -> BMP_280/4(P_ref)
  BMP_280/1(BaroAlt) -> Bus Creator/17  "quota_baro"
  Demux1/5 -> Bus Creator/12  "q"
  In4/1 -> Bus Creator/21  "PWM_autopilota"
  [mario] -> Bus Creator/20  "mario"
  P_int/1 -> BMP_280/3(P_int)
  Demux1/3 -> Bus Creator/10  "acc z"
  Bus Creator/1 -> In_filtro/1
  Demux/5 -> Bus Creator/5  "heading"
  Comandi/1 -> Bus Creator/7  "Comandi"
  Demux1/4 -> Bus Creator/11  "p"
  Data Type Conversion1/1 -> Manual Switch1/2
  Demux/4 -> Bus Creator/4  "quota_GPS"
  Demux1/1 -> Bus Creator/8  "acc x"
  Cal_Alt/1 -> GPS_Venus/1(Cal_alt), BMP_280/1(Cal_Alt)
  Demux/1 -> Bus Creator/1  "Lat"
  Demux1/7 -> Bus Creator/14  "phi"
  Demux1/2 -> Bus Creator/9  "acc y"
  Demux1/9 -> Bus Creator/16  "psi"
  MTi/1(Misure MTi) -> Data Type Conversion1/1
  Demux/2 -> Bus Creator/2  "Long"
  Constant/1 -> attopilot_mis/1
  Demux1/6 -> Bus Creator/13  "r"
  T_0/1 -> BMP_280/2(T_0)
  Demux/3 -> Bus Creator/3  "V_GPS"
  Manual Switch/1 -> Demux/1
  Constant8/1 -> Manual Switch/2
  Constant1/1 -> Manual Switch1/1
  Manual Switch1/1 -> Demux1/1
  BMP_280/2(P_refer) -> P_refer/1
  BMP_280/3(P_RAW) -> P_RAW/1, Bus Creator/18  "pressione"
  BMP_280/4(AB_T) -> Bus Creator/19, AB_T/1  "temperatura"
  BMP_280/5(T_0_out) -> T_0_out/1
  Constant9/1 -> [mario]
  Counter Limited/1 -> Compare To Constant/1
  Compare To Constant/1 -> S-Function Builder/1
  Pitot_Lidar/1(velocity) -> Manual Switch2/1  "V_pitot"
  Manual Switch2/1 -> Bus Creator/22  "V_pitot"
  Constant2/1 -> Manual Switch2/2
  Constant3/1 -> Manual Switch3/2
  Manual Switch3/1 -> Bus Creator/23  "dist_lidar"
  Pitot_Lidar/2(distance) -> Manual Switch3/1  "dist_lidar"
  Pitot_Lidar/3(dp) -> dp/1
  registro memoria2 13/1 -> Byte Unpack/1
  Byte Unpack/1 -> pwm_min_max/1

== system Aenea_model/AUTOPILOT_MODEL/PARAMETRI SISTEMA DI CONTROLLO ==
  Tas : Inport
  Bus Creator1 : BusCreator  Inputs=19
  Gain3 : Gain  Gain=-1
  K AntiWindup-Bumpless AP quota : Constant  Value=K_AW_B_AP_quota  OutDataTypeStr=int16
  K AntiWindup-Bumpless controllore beccheggio : Constant  Value=K_AW_B_becc  OutDataTypeStr=single
  K AntiWindup-Bumpless controllore imbardata : Constant  Value=K_AW_B_imb  OutDataTypeStr=int8
  K AntiWindup-Bumpless controllore rollio : Constant  Value=K_AW_B_roll  OutDataTypeStr=int16
  K AntiWindup-Bumpless controllore rollio1 : Constant  Commented=on  Value=500  OutDataTypeStr=int16
  K controllo imbardata inversa : Constant  Value=K_imb_inv  OutDataTypeStr=int8
  Ki AP quota Select : Constant  Value=Ki_AP_quota_select  OutDataTypeStr=single
  Ki AP rotta1 : Constant  Value=Ki_AP_rotta  OutDataTypeStr=single
  Ki AP velocità : Constant  Value=Ki_AP_vel  OutDataTypeStr=single
  Ki controllore  beccheggio1 : Constant  Value=Ki_becch  OutDataTypeStr=single
  Ki controllore  rollio1 : Constant  Commented=on  Value=0.013  OutDataTypeStr=single
  Ki controllore  rollio2 : Constant  Commented=on  Value=0.025  OutDataTypeStr=single
  Ki controllore  rollio3 : Constant  Value=Ki_roll  OutDataTypeStr=single
  Kp AP quota Hold2 : Constant  Commented=on  Value=0.15  OutDataTypeStr=single
  Kp AP quota Select : Constant  Value=Kp_AP_quota_select  OutDataTypeStr=single
  Kp AP rotta : Constant  Value=Kp_AP_rotta  OutDataTypeStr=single
  Kp AP rotta1 : Constant  Commented=on  Value=0.3  OutDataTypeStr=single
  Kp AP velocità : Constant  Value=Kp_AP_vel  OutDataTypeStr=single
  Kp controllore  rollio1 : Constant  Commented=on  Value=0.15  OutDataTypeStr=single
  Kp controllore  rollio2 : Constant  Commented=on  Value=0.13  OutDataTypeStr=single
  Kp controllore  rollio3 : Constant  Value=Kp_roll  OutDataTypeStr=single
  Kp controllore  velocità rollio1 : Constant  Commented=on  Value=0.04  OutDataTypeStr=single
  Kp controllore  velocità rollio2 : Constant  Commented=on  Value=0.05  OutDataTypeStr=single
  Kp controllore  velocità rollio3 : Constant  Value=Kp_p  OutDataTypeStr=single
  Kp controllore beccheggio1 : Constant  Value=Kp_becch  OutDataTypeStr=single
  Kp controllore imbardata : Constant  Value=Kp_imb  OutDataTypeStr=single
  Kp controllore imbardata1 : Constant  Commented=on  Value=-0.1  OutDataTypeStr=single
  Kp controllore velocità beccheggio1 : Constant  Value=Kp_q  OutDataTypeStr=single
  Saturation : Saturate  UpperLimit=Kp_AP_quota_hold_l  LowerLimit=Kp_AP_quota_hold_h
  n-D Lookup Table : Lookup_n-D  NumberOfTableDimensions=1  BreakpointsForDimension1=[V_stall V_max*0.8]  Table=[Kp_AP_quota_hold_l Kp_AP_quota_hold_h]  RndMeth=Simplest  InputSameDT=on
  Parametri Sistema di Controllo : Outport  VectorParamsAs1DForOutWhenUnconnected=off
  wires:
  Gain3/1 -> Bus Creator1/19  "K_imb_inv"
  Bus Creator1/1 -> Parametri Sistema di Controllo/1  "Cond.Volo.Richiesta"
  Kp controllore imbardata/1 -> Bus Creator1/7  "Kp_imb"
  Kp AP velocità/1 -> Bus Creator1/8  "Kp_AP_vel"
  Saturation/1 -> Bus Creator1/10  "Kp_AP_quota_hold"
  Kp AP quota Select/1 -> Bus Creator1/11  "Kp_AP_quota_select"
  Ki AP quota Select/1 -> Bus Creator1/12  "Ki_AP_quota_select"
  Kp AP rotta/1 -> Bus Creator1/13  "Kp_AP_rotta"
  K AntiWindup-Bumpless controllore beccheggio/1 -> Bus Creator1/15  "K_AW-B_becc"
  K AntiWindup-Bumpless controllore rollio/1 -> Bus Creator1/16  "K_AW-B_roll"
  K AntiWindup-Bumpless controllore imbardata/1 -> Bus Creator1/17  "K_AW-B_imb"
  K AntiWindup-Bumpless AP quota/1 -> Bus Creator1/18  "K_AW-B_AP_quota"
  Ki AP velocità/1 -> Bus Creator1/9  "Ki_AP_vel"
  Ki AP rotta1/1 -> Bus Creator1/14  "Ki_AP_rotta"
  Kp controllore  rollio3/1 -> Bus Creator1/4  "Kp_roll"
  Kp controllore  velocità rollio3/1 -> Bus Creator1/6  "Kp_p"
  Ki controllore  rollio3/1 -> Bus Creator1/5  "Ki_roll"
  n-D Lookup Table/1 -> Saturation/1
  Tas/1 -> n-D Lookup Table/1
  Kp controllore beccheggio1/1 -> Bus Creator1/1  "Kp_becch"
  Ki controllore  beccheggio1/1 -> Bus Creator1/2  "Ki_becch"
  Kp controllore velocità beccheggio1/1 -> Bus Creator1/3  "Kp_q"
  K controllo imbardata inversa/1 -> Gain3/1  "K_imb_inv"

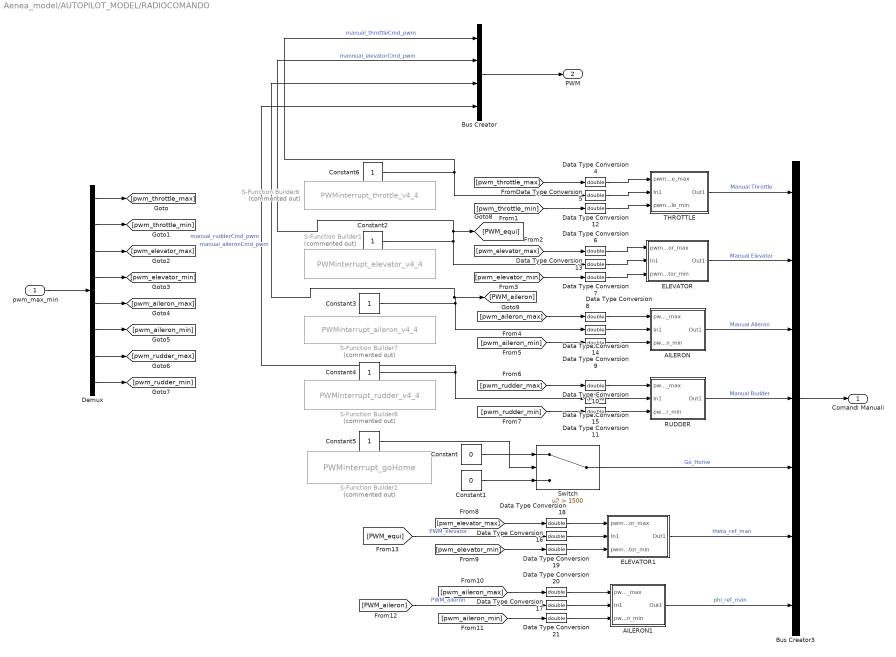
== system Aenea_model/AUTOPILOT_MODEL/RADIOCOMANDO ==
  pwm_max_min : Inport
  AILERON : Subsystem
  AILERON1 : Subsystem
  Bus Creator : BusCreator  Inputs=4
  Bus Creator3 : BusCreator  Inputs=7
  Constant : Constant  Value=0
  Constant1 : Constant  Value=0
  Constant{2..6} (5 alike) : Constant  OutDataTypeStr=int16
  Data Type Conversion{4..21} (18 alike) : DataTypeConversion  OutDataTypeStr=double
  Demux : Demux  Outputs=8
  ELEVATOR : Subsystem
  ELEVATOR1 : Subsystem
  RUDDER : Subsystem
  S-Function Builder1 : S-Function  Commented=on  InitFcn=try, set_param(gcb,'FunctionName','PWMinterrupt_elevator_v4_4'), end  FunctionName=PWMinterrupt_elevator_v4_4  SFunctionModules=PWMinterrupt_elevator_v4_4_wrapper calcInputElevator  SFunctionDeploymentMode=off  EnableBusSupport=off  mask(S-Function Builder){}
      mask init: same as Aenea_model/LOG_DATA_MODEL/S-Function Builder
      settings: CopyFcn=set_param(gcbh,'LinkStatus','none')  PreSaveFcn=try, set_param(gcb,'FunctionName','PWMinterrupt_elevator_v4_4'), end  OpenFcn=sfunctionwizard(gcbh)
      mask Display: plot(val(:,1),val(:,2)),disp(sys),port_label('output',1,'out')
  S-Function Builder2 : S-Function  Commented=on  InitFcn=try, set_param(gcb,'FunctionName','PWMinterrupt_goHome'), end  FunctionName=PWMinterrupt_goHome  SFunctionModules=PWMinterrupt_goHome_wrapper calcInput_go_Home  SFunctionDeploymentMode=off  EnableBusSupport=off  mask(S-Function Builder){}
      mask init: same as Aenea_model/LOG_DATA_MODEL/S-Function Builder
      settings: CopyFcn=set_param(gcbh,'LinkStatus','none')  PreSaveFcn=try, set_param(gcb,'FunctionName','PWMinterrupt_goHome'), end  OpenFcn=sfunctionwizard(gcbh)
      mask Display: plot(val(:,1),val(:,2)),disp(sys),port_label('output',1,'out')
  S-Function Builder6 : S-Function  Commented=on  InitFcn=try, set_param(gcb,'FunctionName','PWMinterrupt_throttle_v4_4'), end  FunctionName=PWMinterrupt_throttle_v4_4  SFunctionModules=PWMinterrupt_throttle_v4_4_wrapper calcInputThrottle  SFunctionDeploymentMode=off  EnableBusSupport=off  mask(S-Function Builder){}
      mask init: same as Aenea_model/LOG_DATA_MODEL/S-Function Builder
      settings: CopyFcn=set_param(gcbh,'LinkStatus','none')  PreSaveFcn=try, set_param(gcb,'FunctionName','PWMinterrupt_throttle_v4_4'), end  OpenFcn=sfunctionwizard(gcbh)
      mask Display: plot(val(:,1),val(:,2)),disp(sys),port_label('output',1,'out')
  S-Function Builder7 : S-Function  Commented=on  InitFcn=try, set_param(gcb,'FunctionName','PWMinterrupt_aileron_v4_4'), end  FunctionName=PWMinterrupt_aileron_v4_4  SFunctionModules=PWMinterrupt_aileron_v4_4_wrapper calcInputAileron  SFunctionDeploymentMode=off  EnableBusSupport=off  mask(S-Function Builder){}
      mask init: same as Aenea_model/LOG_DATA_MODEL/S-Function Builder
      settings: CopyFcn=set_param(gcbh,'LinkStatus','none')  PreSaveFcn=try, set_param(gcb,'FunctionName','PWMinterrupt_aileron_v4_4'), end  OpenFcn=sfunctionwizard(gcbh)
      mask Display: plot(val(:,1),val(:,2)),disp(sys), port_label('output',1,'out')
  S-Function Builder8 : S-Function  Commented=on  InitFcn=try, set_param(gcb,'FunctionName','PWMinterrupt_rudder_v4_4'), end  FunctionName=PWMinterrupt_rudder_v4_4  SFunctionModules=PWMinterrupt_rudder_v4_4_wrapper calcInputRudder  SFunctionDeploymentMode=off  EnableBusSupport=off  mask(S-Function Builder){}
      mask init: same as Aenea_model/LOG_DATA_MODEL/S-Function Builder
      settings: CopyFcn=set_param(gcbh,'LinkStatus','none')  PreSaveFcn=try, set_param(gcb,'FunctionName','PWMinterrupt_rudder_v4_4'), end  OpenFcn=sfunctionwizard(gcbh)
      mask Display: plot(val(:,1),val(:,2)),disp(sys),port_label('output',1,'out')
  Switch : Switch  Criteria=u2 > Threshold  Threshold=1500
  THROTTLE : Subsystem
  Comandi Manuali : Outport  VectorParamsAs1DForOutWhenUnconnected=off
  PWM : Outport  Port=2  VectorParamsAs1DForOutWhenUnconnected=off
  wires:
  Bus Creator3/1 -> Comandi Manuali/1
  Constant5/1 -> Switch/2
  Constant/1 -> Switch/1
  Constant1/1 -> Switch/3
  Switch/1 -> Bus Creator3/5  "Go_Home"
  Constant4/1 -> Bus Creator/4, Data Type Conversion15/1  "manual_rudderCmd_pwm"
  Constant2/1 -> Data Type Conversion13/1, Bus Creator/2, [PWM_equi]  "mannual_elevatorCmd_pwm"
  Constant3/1 -> Data Type Conversion14/1, Bus Creator/3, [PWM_aileron]  "manual_aileronCmd_pwm"
  Constant6/1 -> Bus Creator/1, Data Type Conversion5/1  "manual_throttleCmd_pwm"
  THROTTLE/1(Out1) -> Bus Creator3/1  "Manual Throttle"
  ELEVATOR/1(Out1) -> Bus Creator3/2  "Manual Elevator"
  AILERON/1(Out1) -> Bus Creator3/3  "Manual Aileron"
  RUDDER/1(Out1) -> Bus Creator3/4  "Manual Rudder"
  Bus Creator/1 -> PWM/1
  pwm_max_min/1 -> Demux/1
  Demux/1 -> [pwm_throttle_max]
  Demux/2 -> [pwm_throttle_min]
  Demux/3 -> [pwm_elevator_max]
  Demux/4 -> [pwm_elevator_min]
  Demux/5 -> [pwm_aileron_max]
  Demux/6 -> [pwm_aileron_min]
  Demux/8 -> [pwm_rudder_min]
  Demux/7 -> [pwm_rudder_max]
  [pwm_elevator_min] -> Data Type Conversion7/1
  [pwm_elevator_max] -> Data Type Conversion6/1
  [pwm_aileron_min] -> Data Type Conversion9/1
  [pwm_aileron_max] -> Data Type Conversion8/1
  [pwm_rudder_max] -> Data Type Conversion10/1
  [pwm_rudder_min] -> Data Type Conversion11/1
  [pwm_throttle_max] -> Data Type Conversion4/1
  [pwm_throttle_min] -> Data Type Conversion12/1
  Data Type Conversion6/1 -> ELEVATOR/1(pwm_elevator_max)
  Data Type Conversion7/1 -> ELEVATOR/3(pwm_elevator_min)
  Data Type Conversion8/1 -> AILERON/1(pwm_aileron_max)
  Data Type Conversion9/1 -> AILERON/3(pwm_aileron_min)
  Data Type Conversion10/1 -> RUDDER/1(pwm_rudder_max)
  Data Type Conversion11/1 -> RUDDER/3(pwm_rudder_min)
  Data Type Conversion4/1 -> THROTTLE/1(pwm_throttle_max)
  Data Type Conversion5/1 -> THROTTLE/2(In1)
  Data Type Conversion12/1 -> THROTTLE/3(pwm_throttle_min)
  Data Type Conversion13/1 -> ELEVATOR/2(In1)
  Data Type Conversion14/1 -> AILERON/2(In1)
  Data Type Conversion15/1 -> RUDDER/2(In1)
  [pwm_aileron_max] -> Data Type Conversion20/1
  AILERON1/1(Out1) -> Bus Creator3/7  "phi_ref_man"
  [PWM_equi] -> Data Type Conversion16/1  "PWM_elevator"
  ELEVATOR1/1(Out1) -> Bus Creator3/6  "theta_ref_man"
  [pwm_elevator_min] -> Data Type Conversion19/1
  Data Type Conversion17/1 -> AILERON1/2(In1)
  [pwm_aileron_min] -> Data Type Conversion21/1
  Data Type Conversion21/1 -> AILERON1/3(pwm_aileron_min)
  Data Type Conversion18/1 -> ELEVATOR1/1(pwm_elevator_max)
  Data Type Conversion16/1 -> ELEVATOR1/2(In1)
  Data Type Conversion20/1 -> AILERON1/1(pwm_aileron_max)
  Data Type Conversion19/1 -> ELEVATOR1/3(pwm_elevator_min)
  [pwm_elevator_max] -> Data Type Conversion18/1
  [PWM_aileron] -> Data Type Conversion17/1  "PWM_aileron"
